simulink model "currentController"  (R2025b)
settings: Solver=FixedStepDiscrete  StartTime=0.0  StopTime=10.0  FixedStep=1e-3/8  RelTol=1e-3
undefined symbols (not defined in the file or in its folder): controller_mode, controller_modes, NumBits1, NumBits2, Slope1, Slope2
libraries: simulink x2
settings Model: DataDictionary=motorData.sldd  Creator=karadeli  LastModifiedBy=karadeli
settings OptimizationCC: DefaultParameterBehavior=Inlined  GainParamInheritBuiltInType=on  UseFloatMulNetSlope=on  DefaultUnderspecifiedDataType=single  InlineInvariantSignals=on  PassReuseOutputArgsAs=Individual arguments  ZeroExternalMemoryAtStartup=off  ZeroInternalMemoryAtStartup=off  NoFixptDivByZeroProtection=on  EfficientFloat2IntCast=on  LifeSpan=1  OptimizeBlockOrder=speed  DifferentSizesBufferReuse=on  EfficientTunableParamExpr=on
settings DebuggingCC: ParamSuppressDoubleToSinglePrecisionLossMsg=on  ParameterTunabilityLossMsg=error  AllowSymbolicDim=off
settings HardwareCC: ProdBitPerPointer=32.0  ProdBitPerSizeT=32.0  ProdBitPerPtrDiffT=32.0  ProdLargestAtomicInteger=Long  ProdLargestAtomicFloat=Double  ProdWordSize=32.0  ProdLongLongMode=on  ProdHWDeviceType=ARM Compatible->ARM Cortex-M  TargetLargestAtomicInteger=Long  TargetLargestAtomicFloat=Double  TargetIntDivRoundTo=Zero  TargetEndianess=LittleEndian  TargetHWDeviceType=ARM Compatible->ARM Cortex-M
settings SFSimCC: MATLABDynamicMemAlloc=off
settings RTWCC: SystemTargetFile=ert.tlc  GenCodeOnly=on  TemplateMakefile=ert_default_tmf  TargetLang=C++  Description=Embedded Coder
settings CodeAppCC: ForceParamTrailComments=on  IgnoreCustomStorageClasses=off  OperatorAnnotations=on  SimulinkDataObjDesc=on  SFDataObjDesc=on  CustomSymbolStrGlobalVar=rt$N$M  CustomSymbolStrType=$N$M  CustomSymbolStrFcn=$N$M$F  CustomSymbolStrMacro=$N$M  InsertBlockDesc=on
settings ERTTargetCC: RootIOFormat=Structure reference  ERTCustomFileTemplate=example_file_process.tlc  ERTFilePackagingFormat=CompactWithDataFile  TargetLangStandard=C++11 (ISO)  GenerateSampleERTMain=on  IncludeMdlTerminateFcn=off  CombineSignalStateStructs=on  SuppressErrorStatus=on  SupportAbsoluteTime=off  CodeInterfacePackaging=C++ class  SubcomponentCodeInterfacePackaging=C++ class  SupportComplex=off  SupportNonInlinedSFcns=on  RemoveDisableFunc=on

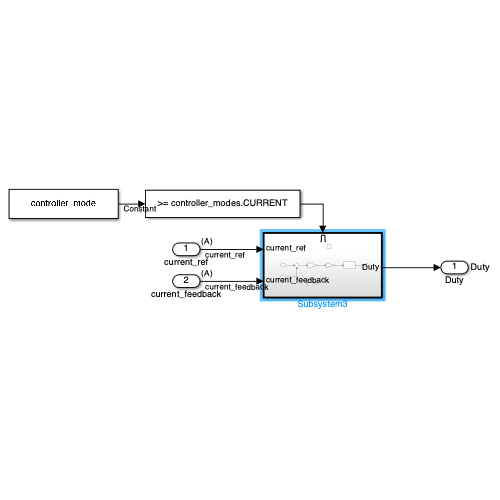
[thumbnail: Simulink's stored preview of the top-level diagram]
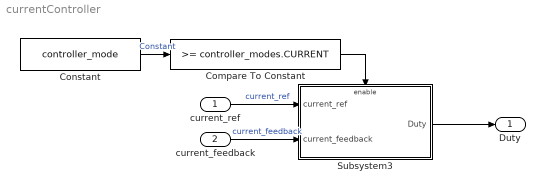
== system currentController ==
  current_ref : Inport  Unit=A  Interpolate=off
  current_feedback : Inport  Port=2  Unit=A  Interpolate=off
  Compare To Constant : simulink/Logic and Bit Operations/Compare To Constant  relop=>=  const=controller_modes.CURRENT  OutDataTypeStr=boolean
  Constant : Constant  Value=controller_mode  SampleTime=-1
  Subsystem3 : Subsystem
  Duty : Outport  SignalName=Duty
  wires:
  current_feedback/1 -> Subsystem3/2(current_feedback)  "current_feedback"
  current_ref/1 -> Subsystem3/1(current_ref)  "current_ref"
  Constant/1 -> Compare To Constant/1  "Constant"
  Subsystem3/1(Duty) -> Duty/1
  Compare To Constant/1 -> Subsystem3/Enable

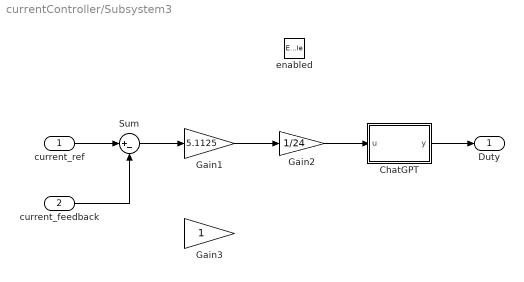
== system currentController/Subsystem3 ==
  current_ref : Inport
  current_feedback : Inport  Port=2
  enabled : EnablePort  StatesWhenEnabling=reset
  ChatGPT : Subsystem  AncestorBlock=simulink/Discrete/Transfer Fcn Lead or Lag  mask(Lead or Lag Compensator){PoleZ=0.9999, ZeroZ=0.522, ICPrevOutput=0.0, ICPrevInput=0.0, RndMeth=Floor, DoSatur=off}
      mask prompts: PoleZ "Simulink:masks:PoleOfCompensatorinZPlane_MP"; ZeroZ "Simulink:masks:ZeroOfCompensatorinZPlane_MP"; ICPrevOutput "Simulink:masks:InitialConditionForPreviousOutput_MP"; ICPrevInput "Simulink:masks:InitialConditionForPreviousInput_MP"; RndMeth "Simulink:masks:IntegerRoundingMode_MP"; DoSatur "Simulink:masks:SaturateToMaxOrMinWhenOverflowsOccur_MP"
      mask help: Simulink:masks:LeadOrLagCompensator_MD
      mask init:
      | if ((PoleZ < 0) || (PoleZ >= 1))
      |    error('Pole position must be a positive number less than 1')
      | end
      | if ((ZeroZ < 0) || (ZeroZ > 1))
      |    error('Zero position must be a positive number less than or equal to 1')
      | end
      | blkH = gcbh;
      | blkName = getfullname(blkH);
      | 
      | vRndMeth = get_param(blkH,'RndMeth');
      | vDoSatur = get_param(blkH,'DoSatur');
      | DCGain = (1-ZeroZ)./(1-PoleZ);
      | maxGain = max( 1, max(max(abs(DCGain))) );
      | OutputSlopeMult = 2^ceil(log2(maxGain));
      | OutputSlopeMult = double(OutputSlopeMult);
      | % SlopeMult is a non-tunable parameter and so do not change it while simulation is running
      | if (~strcmp(get_param(bdroot(blkH), 'SimulationStatus'), 'running') && ~strcmp(get_param(bdroot(blkH), 'SimulationStatus'), 'paused'))
      |     set_param([blkName '/DataTypeProp'], 'SlopeMult', num2str(OutputSlopeMult));
      | end
      | set_param([blkName,'/GainZero'],'RndMeth',vRndMeth, ...
      | 	'DoSatur',vDoSatur);
      | set_param([blkName,'/GainPole'],'RndMeth',vRndMeth, ...
      | 	'DoSatur',vDoSatur);
      | set_param([blkName,'/Downcast'],'RndMeth',vRndMeth, ...
      | 	'DoSatur',vDoSatur);
      | set_param([blkName,'/Sum'],'RndMeth',vRndMeth, ...
      | 	'DoSatur',vDoSatur);
      mask TypeOptions RndMeth: Simulink:masks:Ceiling | Simulink:masks:Convergent | Simulink:masks:Floor | Simulink:masks:Nearest | Simulink:masks:Round | Simulink:masks:Simplest | Simulink:masks:Zero
      mask Display: dpoly([1 -ZeroZ],[1 -PoleZ],'z')
  Gain1 : Gain  Gain=5.1125
  Gain2 : Gain  Gain=1/24
  Gain3 : Gain
  Sum : Sum  Inputs=|+-
  Duty : Outport  OutputWhenDisabled=reset  InitialOutput=0
  wires:
  ChatGPT/1(y) -> Duty/1
  current_feedback/1 -> Sum/2
  current_ref/1 -> Sum/1
  Gain2/1 -> ChatGPT/1(u)
  Sum/1 -> Gain1/1
  Gain1/1 -> Gain2/1

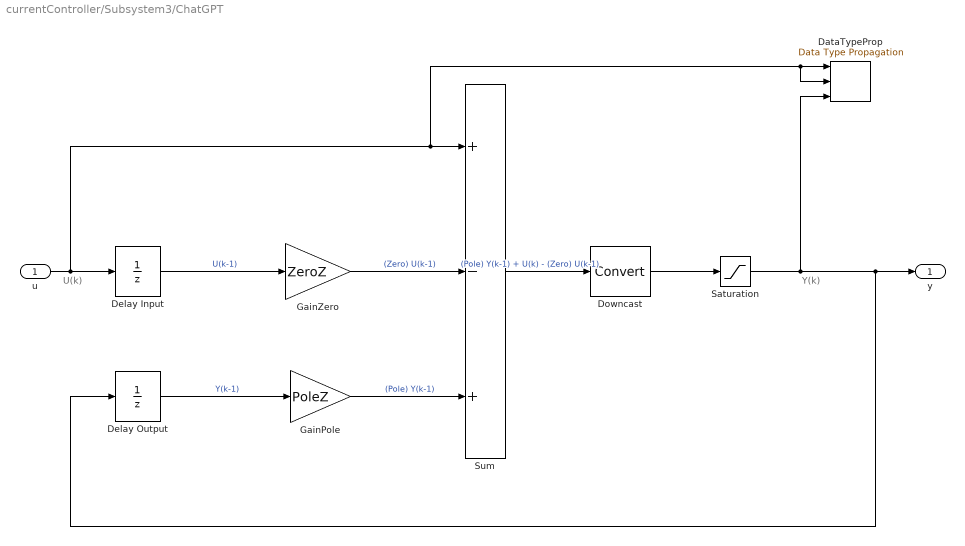
== system currentController/Subsystem3/ChatGPT ==
  note: U(k)
  note: Y(k)
  u : Inport
  DataTypeProp : simulink/Signal Attributes/Data Type Propagation  PropDataType=fixdt(1, 16)  IfRefDouble=double  IfRefSingle=single  IsSigned=IsSigned1 or IsSigned2  NumBitsBase=max([NumBits1 NumBits2])  NumBitsMult=1  NumBitsAdd=0  NumBitsAllowFinal=-1  PropScaling=2^-10  ValuesUsedBestPrec=[5 -7]  SlopeBase=min([Slope1 Slope2])  SlopeMult=8192  SlopeAdd=0  BiasBase=Bias1  BiasMult=0  BiasAdd=0
  Delay Input : UnitDelay  Description=Store in Global RAM  DisableCoverage=on  InitialCondition=ICPrevInput  SampleTime=-1  HasFrameUpgradeWarning=on
      settings: AttributesFormatString=%<Description>
  Delay Output : UnitDelay  Description=Store in Global RAM  DisableCoverage=on  InitialCondition=ICPrevOutput  SampleTime=-1  HasFrameUpgradeWarning=on
      settings: AttributesFormatString=%<Description>
  Downcast : DataTypeConversion  Description=|  SaturateOnIntegerOverflow=off  RndMeth=Floor  LockScale=on
      | Reduce from CPU Size
      |  to Global RAM Size
      settings: AttributesFormatString=%<Description>
  GainPole : Gain  Description=Multiply in CPU  DisableCoverage=on  Gain=PoleZ  LockScale=on
      settings: AttributesFormatString=%<Description>
  GainZero : Gain  Description=Multiply in CPU  DisableCoverage=on  Gain=ZeroZ  LockScale=on
      settings: AttributesFormatString=%<Description>
  Saturation : Saturate  UpperLimit=1  LowerLimit=-1
  Sum : Sum  Description=Add in CPU  DisableCoverage=on  Inputs=+-+  LockScale=on
      settings: AttributesFormatString=%<Description>
  y : Outport  InitialOutput=0
  wires:
  Downcast/1 -> Saturation/1
  Sum/1 -> Downcast/1  "(Pole) Y(k-1) + U(k) - (Zero) U(k-1)"
  GainPole/1 -> Sum/3  "(Pole) Y(k-1)"
  GainZero/1 -> Sum/2  "(Zero) U(k-1)"
  Delay Input/1 -> GainZero/1  "U(k-1)"
  Delay Output/1 -> GainPole/1  "Y(k-1)"
  u/1 -> Delay Input/1, Sum/1, DataTypeProp/1, DataTypeProp/2
  Saturation/1 -> DataTypeProp/3, Delay Output/1, y/1
